simulink model "ROPOD_4Wheel_kinb_cntr"  (R2017b)
settings: Solver=FixedStepAuto  StartTime=0.0  StopTime=Inf  FixedStep=Ts  RelTol=1e-3
PreLoadFcn:
  | init_model
InitFcn:
  | init_model
values from neighbouring files (symbols this model uses):
  max_ropod_acc_theta = pi/16    (= 0.196349540849)    [init_model.m]
  max_ropod_acc_xy = 1.0    (= 1)    [init_model.m]
  max_ropod_vel_theta = pi/4    (= 0.785398163397)    [init_model.m]
  max_ropod_vel_xy = 1.5    [init_model.m]
  max_sw_current = 10    [init_model.m]
  Nwheels = 4    [init_model.m]
  pivot_offs_sws = [1.0998 0.2956 3.507 0.3641]    [init_model.m]
  SW_COM1_ENABLE1 = hex2dec('0001')    [init_model.m]
  SW_COM1_ENABLE2 = hex2dec('0002')    [init_model.m]
  SW_COM1_MODE_VELOCITY = bitshift(hex2dec('0002'),2)    [init_model.m]
  SW_COM1_USE_TS = hex2dec('8000')    [init_model.m]
  Ts = 0.001    [init_model.m]
  Tsp = 1    [init_model.m]
undefined symbols (not defined in the file or in its folder): Angular, CW1_1, CW1_2, CW1_3, CW1_4, CW2_1, CW2_2, CW2_3, CW2_4, d_w, DiscIntNeverNeededParam, Linear, Pose, ropod_kinmodel_param, rW1_1, rW1_2, rW1_3, rW1_4, rW2_1, rW2_2, rW2_3, rW2_4, s_w, Twist
libraries: robotlib x65, simulink x10, SOEM_EtherCAT_Lib x5, robotcorelib x1
(part 1 of 2)
PreSaveFcn:
  | init_model
settings Model: Creator=cesar  LastModifiedBy=cesar
settings OptimizationCC: PassReuseOutputArgsAs=Individual arguments  MaxStackSize=64
settings DebuggingCC: ParameterTunabilityLossMsg=error
settings HardwareCC: ProdBitPerLong=64  ProdHWDeviceType=Intel->x86-64 (Linux 64)  TargetBitPerLong=64  TargetBitPerPointer=64  TargetBitPerSizeT=64  TargetBitPerPtrDiffT=64  TargetLargestAtomicFloat=Float  TargetIntDivRoundTo=Zero  TargetEndianess=LittleEndian  TargetWordSize=64  TargetHWDeviceType=Intel->x86-64 (Linux 64)
settings SFSimCC: MATLABDynamicMemAlloc=off
settings RTWCC: SystemTargetFile=ert.tlc  HardwareBoard=Robot Operating System (ROS)  TemplateMakefile=ert_default_tmf  GenerateReport=on  RTWVerbose=off  CustomInclude=/usr/local/include/soem  CustomLibrary=/usr/local/lib/libsoem.so  Toolchain=Catkin  BuildConfiguration=Faster Runs  IncludeHyperlinkInReport=on  LaunchReport=on  TargetLang=C++  GenerateTraceInfo=on  GenerateTraceReport=on  GenerateTraceReportSl=on  GenerateTraceReportSf=on  GenerateTraceReportEml=on
settings CodeAppCC: ForceParamTrailComments=on  IgnoreCustomStorageClasses=off  OperatorAnnotations=on  SimulinkDataObjDesc=on  SFDataObjDesc=on  InsertBlockDesc=on
settings ERTTargetCC: SupportNonInlinedSFcns=on

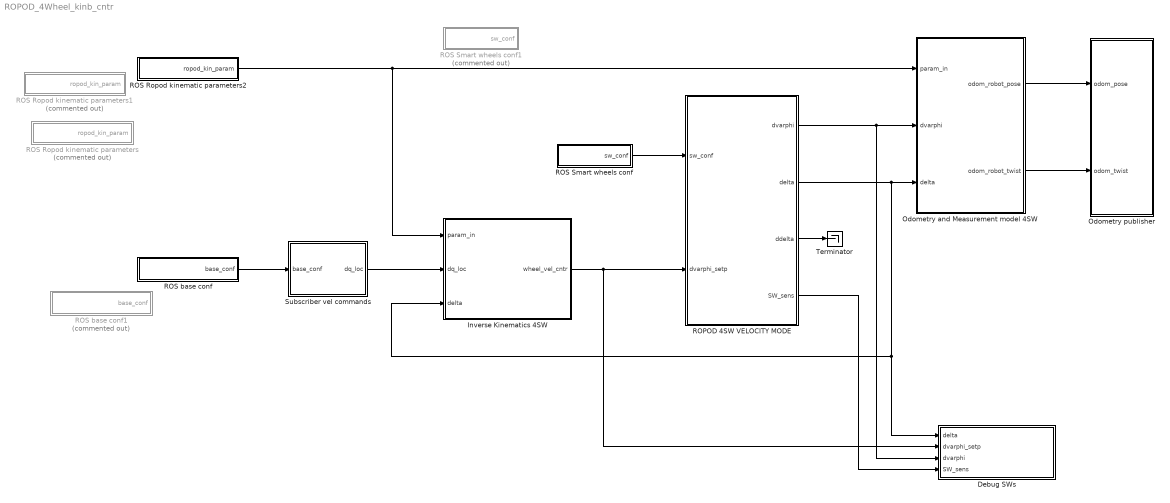
== system ROPOD_4Wheel_kinb_cntr ==
  Debug SWs : Subsystem
  Inverse Kinematics 4SW : Subsystem
  Odometry and Measurement model 4SW : Subsystem
  Odometry publisher : Subsystem
  ROPOD 4SW VELOCITY MODE : Subsystem
  ROS Ropod kinematic parameters : Subsystem  Commented=on
  ROS Ropod kinematic parameters1 : Subsystem  Commented=on
  ROS Ropod kinematic parameters2 : Subsystem
  ROS Smart wheels conf : Subsystem
  ROS Smart wheels conf1 : Subsystem  Commented=on
  ROS base conf : Subsystem
  ROS base conf1 : Subsystem  Commented=on
  Subscriber vel commands : Subsystem
  Terminator : Terminator
  wires:
  ROS Smart wheels conf/1(sw_conf) -> ROPOD 4SW VELOCITY MODE/1(sw_conf)
  ROS Ropod kinematic parameters2/1(ropod_kin_param) -> Inverse Kinematics 4SW/1(param_in), Odometry and Measurement model 4SW/1(param_in)
  Inverse Kinematics 4SW/1(wheel_vel_cntr) -> ROPOD 4SW VELOCITY MODE/2(dvarphi_setp), Debug SWs/2(dvarphi_setp)
  Odometry and Measurement model 4SW/1(odom_robot_pose) -> Odometry publisher/1(odom_pose)
  Odometry and Measurement model 4SW/2(odom_robot_twist) -> Odometry publisher/2(odom_twist)
  Subscriber vel commands/1(dq_loc) -> Inverse Kinematics 4SW/2(dq_loc)
  ROS base conf/1(base_conf) -> Subscriber vel commands/1(base_conf)
  ROPOD 4SW VELOCITY MODE/3(ddelta) -> Terminator/1
  ROPOD 4SW VELOCITY MODE/1(dvarphi) -> Odometry and Measurement model 4SW/2(dvarphi), Debug SWs/3(dvarphi)
  ROPOD 4SW VELOCITY MODE/2(delta) -> Inverse Kinematics 4SW/3(delta), Debug SWs/1(delta), Odometry and Measurement model 4SW/3(delta)
  ROPOD 4SW VELOCITY MODE/4(SW_sens) -> Debug SWs/4(SW_sens)

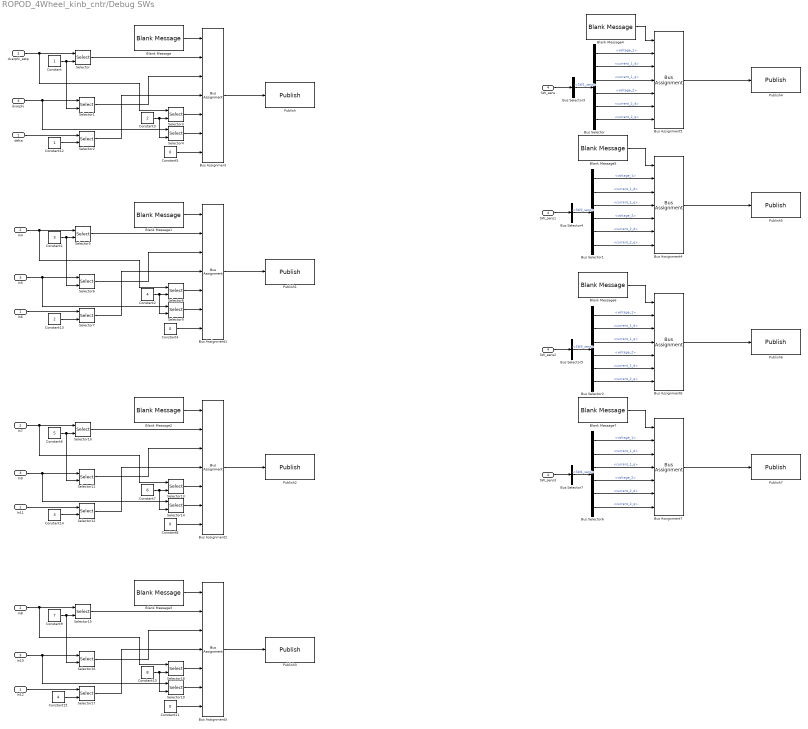
== system ROPOD_4Wheel_kinb_cntr/Debug SWs ==
  delta : Inport
  dvarphi_setp : Inport  Port=2
  dvarphi : Inport  Port=3
  SW_sens : Inport  Port=4
  Blank Message{,1..7} (8 alike) : robotlib/Blank Message  SourceLibraryInfo=This block requires Robotics System Toolbox  messageType=geometry_msgs/Twist  SampleTime=-1
      settings: SourceProductBaseCode=RO
  Bus Assignment{,1..7} (8 alike) : BusAssignment  AssignedSignals=Linear.X,Linear.Y,Linear.Z,Angular.X,Angular.Y,Angular.Z
  Bus Selector{,1..2,6} (4 alike) : BusSelector  OutputSignals=voltage_1,current_1_d,current_1_q,voltage_2,current_2_d,current_2_q
  Bus Selector3 : BusSelector  OutputSignals=SW1_sens
  Bus Selector4 : BusSelector  OutputSignals=SW2_sens
  Bus Selector5 : BusSelector  OutputSignals=SW3_sens
  Bus Selector7 : BusSelector  OutputSignals=SW4_sens
  Constant : Constant
  Constant1 : Constant  Value=3
  Constant10 : Constant  Value=8
  Constant{4..5,8,11} (4 alike) : Constant  Value=0
  Constant12 : Constant
  Constant13 : Constant  Value=2
  Constant14 : Constant  Value=3
  Constant15 : Constant  Value=4
  Constant2 : Constant  Value=4
  Constant3 : Constant  Value=2
  Constant6 : Constant  Value=5
  Constant7 : Constant  Value=6
  Constant9 : Constant  Value=7
  In10 : InportShadow  Port=3
  In11 : InportShadow
  In12 : InportShadow
  In4 : InportShadow  Port=2
  In5 : InportShadow  Port=3
  In6 : InportShadow
  In7 : InportShadow  Port=2
  In8 : InportShadow  Port=2
  In9 : InportShadow  Port=3
  Publish : robotlib/Publish  SourceLibraryInfo=This block requires Robotics System Toolbox  topicSource=Specify your own  topic=/smartw1_debug  messageType=geometry_msgs/Twist  messageQueueLength=1
      settings: SourceProductBaseCode=RO
  Publish1 : robotlib/Publish  SourceLibraryInfo=This block requires Robotics System Toolbox  topicSource=Specify your own  topic=/smartw2_debug  messageType=geometry_msgs/Twist  messageQueueLength=1
      settings: SourceProductBaseCode=RO
  Publish2 : robotlib/Publish  SourceLibraryInfo=This block requires Robotics System Toolbox  topicSource=Specify your own  topic=/smartw3_debug  messageType=geometry_msgs/Twist  messageQueueLength=1
      settings: SourceProductBaseCode=RO
  Publish3 : robotlib/Publish  SourceLibraryInfo=This block requires Robotics System Toolbox  topicSource=Specify your own  topic=/smartw4_debug  messageType=geometry_msgs/Twist  messageQueueLength=1
      settings: SourceProductBaseCode=RO
  Publish4 : robotlib/Publish  SourceLibraryInfo=This block requires Robotics System Toolbox  topicSource=Specify your own  topic=/smartw1_volcurr_debug  messageType=geometry_msgs/Twist  messageQueueLength=1
      settings: SourceProductBaseCode=RO
  Publish5 : robotlib/Publish  SourceLibraryInfo=This block requires Robotics System Toolbox  topicSource=Specify your own  topic=/smartw2_volcurr_debug  messageType=geometry_msgs/Twist  messageQueueLength=1
      settings: SourceProductBaseCode=RO
  Publish6 : robotlib/Publish  SourceLibraryInfo=This block requires Robotics System Toolbox  topicSource=Specify your own  topic=/smartw3_volcurr_debug  messageType=geometry_msgs/Twist  messageQueueLength=1
      settings: SourceProductBaseCode=RO
  Publish7 : robotlib/Publish  SourceLibraryInfo=This block requires Robotics System Toolbox  topicSource=Specify your own  topic=/smartw4_volcurr_debug  messageType=geometry_msgs/Twist  messageQueueLength=1
      settings: SourceProductBaseCode=RO
  SW_sens1 : InportShadow  Port=4
  SW_sens2 : InportShadow  Port=4
  SW_sens3 : InportShadow  Port=4
  Selector{,1,3..6,8..11,13..16,18..19} (16 alike) : Selector  InputPortWidth=8  IndexOptions=Index vector (port)  Indices=[1 3]  OutputSizes=1
  Selector{2,7,12,17} (4 alike) : Selector  InputPortWidth=4  IndexOptions=Index vector (port)  Indices=[1 3]  OutputSizes=1
  wires:
  delta/1 -> Selector2/1
  Constant5/1 -> Bus Assignment/7
  Selector2/1 -> Bus Assignment/4
  Selector3/1 -> Bus Assignment/5
  Constant/1 -> Selector1/2, Selector/2
  Blank Message/1 -> Bus Assignment/1
  Constant3/1 -> Selector4/2, Selector3/2
  Selector/1 -> Bus Assignment/2
  Selector1/1 -> Bus Assignment/3
  dvarphi/1 -> Selector4/1, Selector1/1
  Selector4/1 -> Bus Assignment/6
  dvarphi_setp/1 -> Selector3/1, Selector/1
  Bus Assignment/1 -> Publish/1
  Selector5/1 -> Bus Assignment1/2
  Blank Message1/1 -> Bus Assignment1/1
  Bus Assignment1/1 -> Publish1/1
  Selector7/1 -> Bus Assignment1/4
  In6/1 -> Selector7/1
  Constant2/1 -> Selector9/2, Selector8/2
  Constant1/1 -> Selector6/2, Selector5/2
  Selector8/1 -> Bus Assignment1/5
  Constant4/1 -> Bus Assignment1/7
  Selector6/1 -> Bus Assignment1/3
  Selector9/1 -> Bus Assignment1/6
  In4/1 -> Selector8/1, Selector5/1
  In5/1 -> Selector9/1, Selector6/1
  In11/1 -> Selector12/1
  Selector14/1 -> Bus Assignment2/6
  In9/1 -> Selector14/1, Selector11/1
  Blank Message2/1 -> Bus Assignment2/1
  Selector13/1 -> Bus Assignment2/5
  Constant7/1 -> Selector14/2, Selector13/2
  Selector12/1 -> Bus Assignment2/4
  Selector11/1 -> Bus Assignment2/3
  Constant6/1 -> Selector11/2, Selector10/2
  Bus Assignment2/1 -> Publish2/1
  Selector10/1 -> Bus Assignment2/2
  In7/1 -> Selector13/1, Selector10/1
  Constant8/1 -> Bus Assignment2/7
  In8/1 -> Selector18/1, Selector15/1
  Selector15/1 -> Bus Assignment3/2
  Selector19/1 -> Bus Assignment3/6
  Selector17/1 -> Bus Assignment3/4
  Selector16/1 -> Bus Assignment3/3
  Selector18/1 -> Bus Assignment3/5
  In10/1 -> Selector19/1, Selector16/1
  Constant9/1 -> Selector16/2, Selector15/2
  In12/1 -> Selector17/1
  Constant10/1 -> Selector19/2, Selector18/2
  Blank Message3/1 -> Bus Assignment3/1
  Constant11/1 -> Bus Assignment3/7
  Bus Assignment3/1 -> Publish3/1
  Constant12/1 -> Selector2/2
  Constant13/1 -> Selector7/2
  Constant14/1 -> Selector12/2
  Constant15/1 -> Selector17/2
  Bus Assignment5/1 -> Publish4/1
  Blank Message4/1 -> Bus Assignment5/1
  Bus Selector/2 -> Bus Assignment5/3  "<current_1_d>"
  Bus Selector/1 -> Bus Assignment5/2  "<voltage_1>"
  Bus Selector/3 -> Bus Assignment5/4  "<current_1_q>"
  Bus Selector/4 -> Bus Assignment5/5  "<voltage_2>"
  Bus Selector/5 -> Bus Assignment5/6  "<current_2_d>"
  Bus Selector/6 -> Bus Assignment5/7  "<current_2_q>"
  Bus Assignment4/1 -> Publish5/1
  Bus Selector1/3 -> Bus Assignment4/4  "<current_1_q>"
  Blank Message5/1 -> Bus Assignment4/1
  Bus Selector1/5 -> Bus Assignment4/6  "<current_2_d>"
  Bus Selector1/6 -> Bus Assignment4/7  "<current_2_q>"
  Bus Selector1/4 -> Bus Assignment4/5  "<voltage_2>"
  Bus Selector1/1 -> Bus Assignment4/2  "<voltage_1>"
  Bus Selector1/2 -> Bus Assignment4/3  "<current_1_d>"
  Bus Selector2/5 -> Bus Assignment6/6  "<current_2_d>"
  Bus Selector2/1 -> Bus Assignment6/2  "<voltage_1>"
  Bus Selector2/2 -> Bus Assignment6/3  "<current_1_d>"
  Bus Selector2/4 -> Bus Assignment6/5  "<voltage_2>"
  Bus Selector2/3 -> Bus Assignment6/4  "<current_1_q>"
  Bus Selector2/6 -> Bus Assignment6/7  "<current_2_q>"
  Bus Assignment6/1 -> Publish6/1
  Blank Message6/1 -> Bus Assignment6/1
  SW_sens/1 -> Bus Selector3/1
  Bus Selector3/1 -> Bus Selector/1  "<SW1_sens>"
  Bus Selector4/1 -> Bus Selector1/1  "<SW2_sens>"
  SW_sens1/1 -> Bus Selector4/1
  Bus Selector5/1 -> Bus Selector2/1  "<SW3_sens>"
  SW_sens2/1 -> Bus Selector5/1
  SW_sens3/1 -> Bus Selector7/1
  Bus Selector7/1 -> Bus Selector6/1  "<SW4_sens>"
  Blank Message7/1 -> Bus Assignment7/1
  Bus Assignment7/1 -> Publish7/1
  Bus Selector6/6 -> Bus Assignment7/7  "<current_2_q>"
  Bus Selector6/3 -> Bus Assignment7/4  "<current_1_q>"
  Bus Selector6/4 -> Bus Assignment7/5  "<voltage_2>"
  Bus Selector6/2 -> Bus Assignment7/3  "<current_1_d>"
  Bus Selector6/1 -> Bus Assignment7/2  "<voltage_1>"
  Bus Selector6/5 -> Bus Assignment7/6  "<current_2_d>"

== system ROPOD_4Wheel_kinb_cntr/Inverse Kinematics 4SW ==
  param_in : Inport
  dq_loc : Inport  Port=2
  delta : Inport  Port=3
  Gl_matrix : MATLAB Function  TreatAsAtomicUnit=on
  Product3 : Product  Multiplication=Matrix(*)
  Selector2 : Selector  InputPortWidth=3+3*Nwheels  IndexOptions=Index vector (dialog)  Indices=[3+Nwheels+1:3+3*Nwheels]  OutputSizes=1
  wheel_vel_cntr : Outport
  wires:
  param_in/1 -> Gl_matrix/1(ropod_kinmodel_param_vec)
  Gl_matrix/1(Gl) -> Product3/1
  Product3/1 -> Selector2/1
  delta/1 -> Gl_matrix/2(delta)
  dq_loc/1 -> Product3/2
  Selector2/1 -> wheel_vel_cntr/1

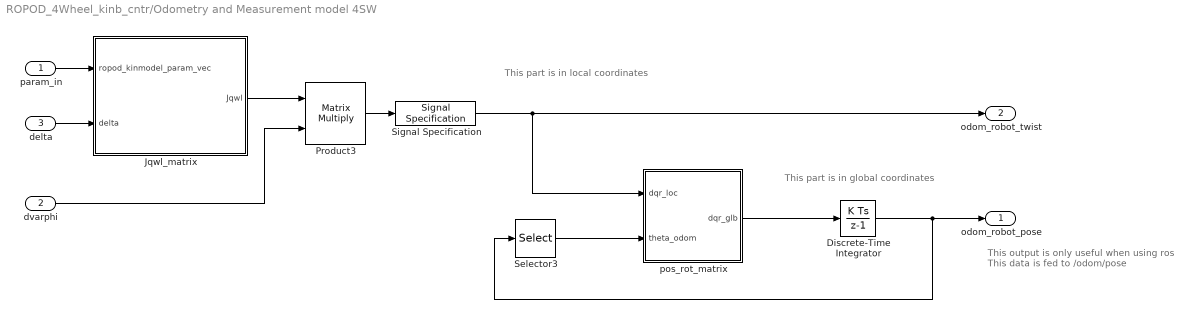
== system ROPOD_4Wheel_kinb_cntr/Odometry and Measurement model 4SW ==
  note: This output is only useful when using ros
      | This data is fed to /odom/pose
  note: This part is in global coordinates
  note: This part is in local coordinates
  param_in : Inport
  dvarphi : Inport  Port=2
  delta : Inport  Port=3
  Discrete-Time Integrator : DiscreteIntegrator  InitialConditionSetting=State (most efficient)  SampleTime=Ts  ICPrevOutput=DiscIntNeverNeededParam  ICPrevScaledInput=DiscIntNeverNeededParam
  Jqwl_matrix : MATLAB Function  TreatAsAtomicUnit=on
  Product3 : Product  Multiplication=Matrix(*)
  Selector3 : Selector  InputPortWidth=3  IndexOptions=Index vector (dialog)  Indices=3  OutputSizes=1
  Signal Specification : SignalSpecification  Dimensions=[3 1]
  pos_rot_matrix : MATLAB Function  TreatAsAtomicUnit=on
  odom_robot_pose : Outport
  odom_robot_twist : Outport  Port=2
  wires:
  Product3/1 -> Signal Specification/1
  param_in/1 -> Jqwl_matrix/1(ropod_kinmodel_param_vec)
  delta/1 -> Jqwl_matrix/2(delta)
  Jqwl_matrix/1(Jqwl) -> Product3/1
  dvarphi/1 -> Product3/2
  Signal Specification/1 -> pos_rot_matrix/1(dqr_loc), odom_robot_twist/1
  Selector3/1 -> pos_rot_matrix/2(theta_odom)
  pos_rot_matrix/1(dqr_glb) -> Discrete-Time Integrator/1
  Discrete-Time Integrator/1 -> odom_robot_pose/1, Selector3/1

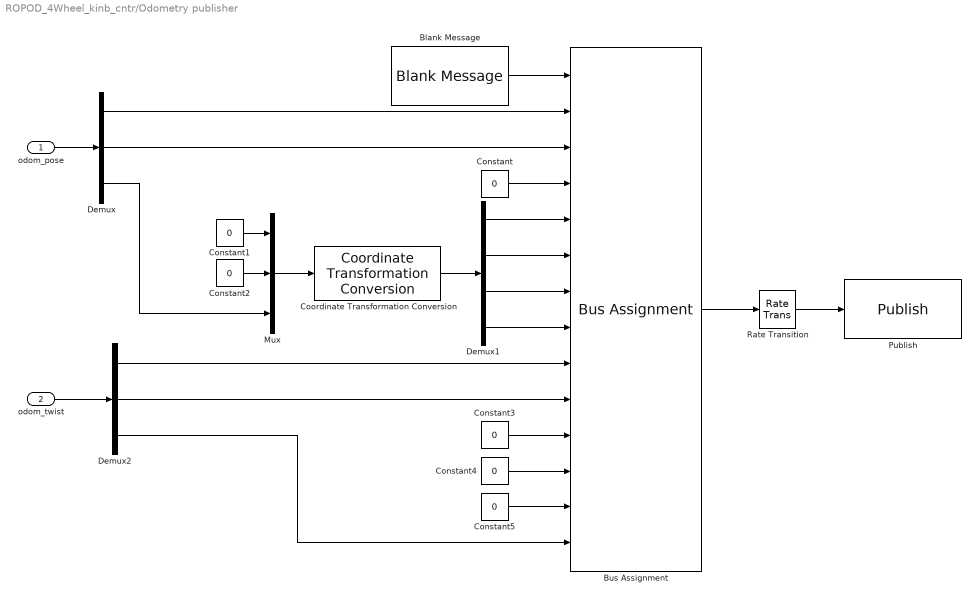
== system ROPOD_4Wheel_kinb_cntr/Odometry publisher ==
  odom_pose : Inport
  odom_twist : Inport  Port=2
  Blank Message : robotlib/Blank Message  SourceLibraryInfo=This block requires Robotics System Toolbox  messageType=nav_msgs/Odometry  SampleTime=-1
      settings: SourceProductBaseCode=RO
  Bus Assignment : BusAssignment  AssignedSignals=Pose.Pose.Position.X,Pose.Pose.Position.Y,Pose.Pose.Position.Z,Pose.Pose.Orientation.X,Pose.Pose.Orientation.Y,Pose.Pose.Orientation.Z,Pose.Pose.Orientation.W,Twist.Twist.Linear.X,Twist.Twist.Linear.Y,Twist.Twist.Linear.Z,Twist.Twist.Angular.X,Twist.Twist.Angular.Y,Twist.Twist.Angular.Z
  Constant{,1..5} (6 alike) : Constant  Value=0
  Coordinate Transformation Conversion : robotcorelib/Coordinate Transformation Conversion  InputRepresentation=Euler Angles  InputEulerSequence=XYZ  ShowTrVecInputPort=on  OutputRepresentation=Quaternion  OutputEulerSequence=ZYX  ShowTrVecOutputPort=on  SimulateUsing=Code generation
      settings: SourceProductBaseCode=RO
  Demux : Demux  Outputs=3
  Demux1 : Demux
  Demux2 : Demux  Outputs=3
  Mux : Mux  Inputs=3
  Publish : robotlib/Publish  SourceLibraryInfo=This block requires Robotics System Toolbox  topicSource=Specify your own  topic=/pico/odom  messageType=nav_msgs/Odometry  messageQueueLength=1
      settings: SourceProductBaseCode=RO
  Rate Transition : RateTransition  OutPortSampleTime=Ts_rost
  wires:
  Demux2/2 -> Bus Assignment/10
  Bus Assignment/1 -> Rate Transition/1
  Constant2/1 -> Mux/2
  Demux1/2 -> Bus Assignment/6
  Constant3/1 -> Bus Assignment/11
  Constant/1 -> Bus Assignment/4
  Constant4/1 -> Bus Assignment/12
  Demux2/1 -> Bus Assignment/9
  Coordinate Transformation Conversion/1 -> Demux1/1
  Constant5/1 -> Bus Assignment/13
  Demux/3 -> Mux/3
  Mux/1 -> Coordinate Transformation Conversion/1
  Demux1/3 -> Bus Assignment/7
  odom_pose/1 -> Demux/1
  Demux1/1 -> Bus Assignment/5
  Demux/1 -> Bus Assignment/2
  Demux1/4 -> Bus Assignment/8
  Constant1/1 -> Mux/1
  odom_twist/1 -> Demux2/1
  Demux/2 -> Bus Assignment/3
  Blank Message/1 -> Bus Assignment/1
  Demux2/3 -> Bus Assignment/14
  Rate Transition/1 -> Publish/1

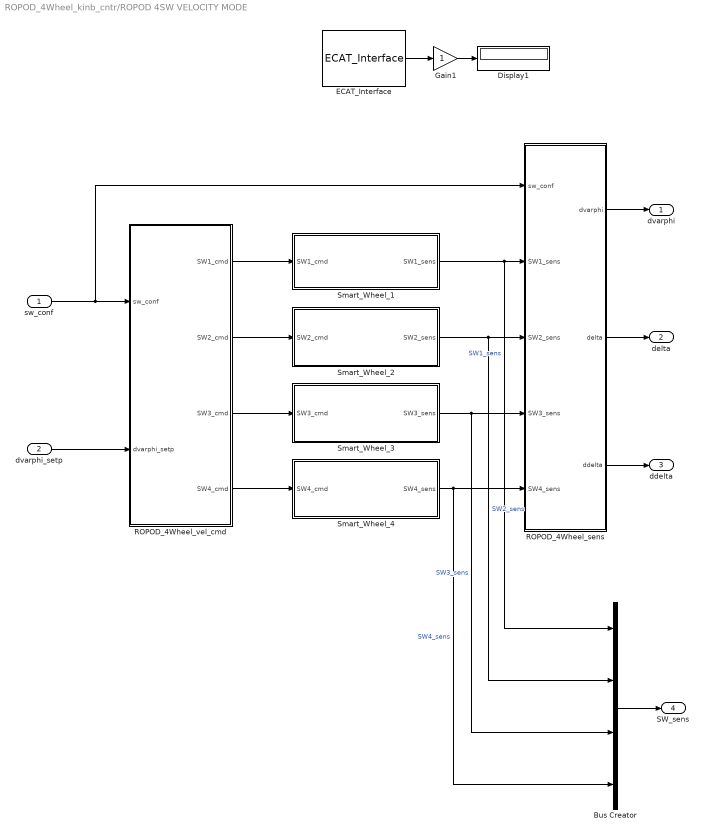
== system ROPOD_4Wheel_kinb_cntr/ROPOD 4SW VELOCITY MODE ==
  sw_conf : Inport
  dvarphi_setp : Inport  Port=2
  Bus Creator : BusCreator  Inputs=4
  Display1 : Display
  ECAT_Interface : SOEM_EtherCAT_Lib/ECAT_Interface  Priority=0  IFINTERFACE=eth0  TS=Ts
      settings: SourceProductName=SOEM_EtherCAT_Lib
  Gain1 : Gain  OutDataTypeStr=double
  ROPOD_4Wheel_sens : Subsystem
  ROPOD_4Wheel_vel_cmd : Subsystem
  Smart_Wheel_1 : Subsystem
  Smart_Wheel_2 : Subsystem
  Smart_Wheel_3 : Subsystem
  Smart_Wheel_4 : Subsystem
  dvarphi : Outport
  delta : Outport  Port=2
  ddelta : Outport  Port=3
  SW_sens : Outport  Port=4
  wires:
  dvarphi_setp/1 -> ROPOD_4Wheel_vel_cmd/2(dvarphi_setp)
  ROPOD_4Wheel_vel_cmd/2(SW2_cmd) -> Smart_Wheel_2/1(SW2_cmd)
  sw_conf/1 -> ROPOD_4Wheel_sens/1(sw_conf), ROPOD_4Wheel_vel_cmd/1(sw_conf)
  ROPOD_4Wheel_vel_cmd/1(SW1_cmd) -> Smart_Wheel_1/1(SW1_cmd)
  Smart_Wheel_1/1(SW1_sens) -> Bus Creator/1, ROPOD_4Wheel_sens/2(SW1_sens)  "SW1_sens"
  ROPOD_4Wheel_sens/2(delta) -> delta/1
  ROPOD_4Wheel_sens/1(dvarphi) -> dvarphi/1
  ECAT_Interface/1 -> Gain1/1
  Gain1/1 -> Display1/1
  ROPOD_4Wheel_vel_cmd/3(SW3_cmd) -> Smart_Wheel_3/1(SW3_cmd)
  ROPOD_4Wheel_sens/3(ddelta) -> ddelta/1
  ROPOD_4Wheel_vel_cmd/4(SW4_cmd) -> Smart_Wheel_4/1(SW4_cmd)
  Smart_Wheel_2/1(SW2_sens) -> Bus Creator/2, ROPOD_4Wheel_sens/3(SW2_sens)  "SW2_sens"
  Smart_Wheel_3/1(SW3_sens) -> Bus Creator/3, ROPOD_4Wheel_sens/4(SW3_sens)  "SW3_sens"
  Smart_Wheel_4/1(SW4_sens) -> Bus Creator/4, ROPOD_4Wheel_sens/5(SW4_sens)  "SW4_sens"
  Bus Creator/1 -> SW_sens/1

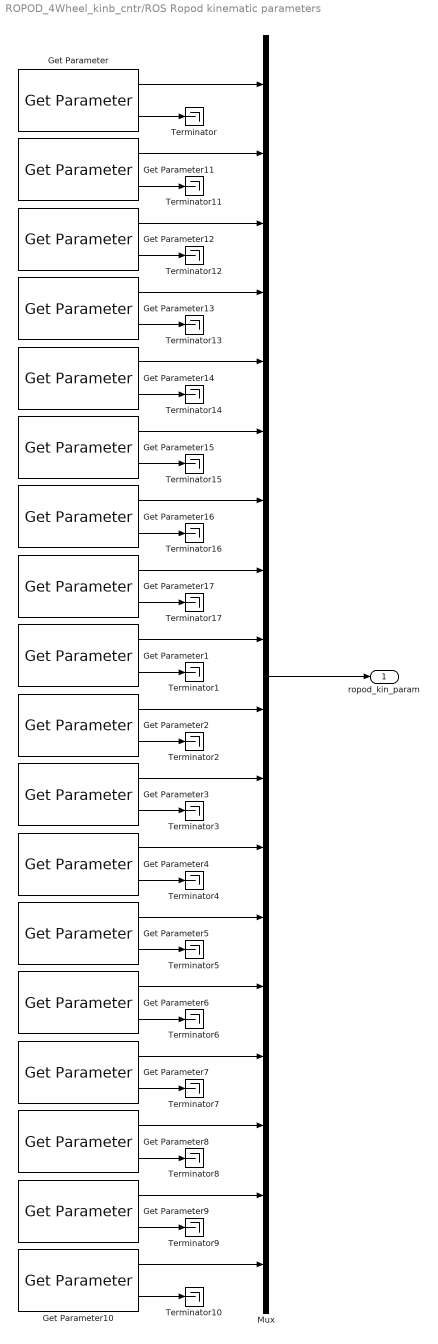
== system ROPOD_4Wheel_kinb_cntr/ROS Ropod kinematic parameters ==
  Get Parameter : robotlib/Get Parameter  SourceLibraryInfo=This block requires Robotics System Toolbox  ParameterSource=Specify your own  ParameterName=/base_kin_model/r_wL_SW1  ParameterType=double  ParameterMaxArrayLength=16  ParameterInitialValue=ropod_kinmodel_param.r_w(1)  SampleTime=-1  ShowErrorCodeOutput=on  ModelName=ROPOD_4Wheel_kinb_cntr  BlockId=ParamGet_ROPOD_4Wheel_kinb_cntr_466
      settings: SourceProductName=Robotics System Toolbox  SourceProductBaseCode=RO
  Get Parameter1 : robotlib/Get Parameter  SourceLibraryInfo=This block requires Robotics System Toolbox  ParameterSource=Specify your own  ParameterName=/base_kin_model/s_w  ParameterType=double  ParameterMaxArrayLength=16  ParameterInitialValue=ropod_kinmodel_param.s_w  SampleTime=-1  ShowErrorCodeOutput=on  ModelName=ROPOD_4Wheel_kinb_cntr  BlockId=ParamGet_ROPOD_4Wheel_kinb_cntr_470
      settings: SourceProductName=Robotics System Toolbox  SourceProductBaseCode=RO
  Get Parameter10 : robotlib/Get Parameter  SourceLibraryInfo=This block requires Robotics System Toolbox  ParameterSource=Specify your own  ParameterName=/base_kin_model/ypos_SW4  ParameterType=double  ParameterMaxArrayLength=16  ParameterInitialValue=ropod_kinmodel_param.C_SW(8)  SampleTime=-1  ShowErrorCodeOutput=on  ModelName=ROPOD_4Wheel_kinb_cntr  BlockId=ParamGet_ROPOD_4Wheel_kinb_cntr_617
      settings: SourceProductName=Robotics System Toolbox  SourceProductBaseCode=RO
  Get Parameter11 : robotlib/Get Parameter  SourceLibraryInfo=This block requires Robotics System Toolbox  ParameterSource=Specify your own  ParameterName=/base_kin_model/r_wR_SW1  ParameterType=double  ParameterMaxArrayLength=16  ParameterInitialValue=ropod_kinmodel_param.r_w(2)  SampleTime=-1  ShowErrorCodeOutput=on  ModelName=ROPOD_4Wheel_kinb_cntr  BlockId=ParamGet_ROPOD_4Wheel_kinb_cntr_648
      settings: SourceProductName=Robotics System Toolbox  SourceProductBaseCode=RO
  Get Parameter12 : robotlib/Get Parameter  SourceLibraryInfo=This block requires Robotics System Toolbox  ParameterSource=Specify your own  ParameterName=/base_kin_model/r_wL_SW2  ParameterType=double  ParameterMaxArrayLength=16  ParameterInitialValue=ropod_kinmodel_param.r_w(3)  SampleTime=-1  ShowErrorCodeOutput=on  ModelName=ROPOD_4Wheel_kinb_cntr  BlockId=ParamGet_ROPOD_4Wheel_kinb_cntr_650
      settings: SourceProductName=Robotics System Toolbox  SourceProductBaseCode=RO
  Get Parameter13 : robotlib/Get Parameter  SourceLibraryInfo=This block requires Robotics System Toolbox  ParameterSource=Specify your own  ParameterName=/base_kin_model/r_wR_SW2  ParameterType=double  ParameterMaxArrayLength=16  ParameterInitialValue=ropod_kinmodel_param.r_w(4)  SampleTime=-1  ShowErrorCodeOutput=on  ModelName=ROPOD_4Wheel_kinb_cntr  BlockId=ParamGet_ROPOD_4Wheel_kinb_cntr_651
      settings: SourceProductName=Robotics System Toolbox  SourceProductBaseCode=RO
  Get Parameter14 : robotlib/Get Parameter  SourceLibraryInfo=This block requires Robotics System Toolbox  ParameterSource=Specify your own  ParameterName=/base_kin_model/r_wL_SW3  ParameterType=double  ParameterMaxArrayLength=16  ParameterInitialValue=ropod_kinmodel_param.r_w(5)  SampleTime=-1  ShowErrorCodeOutput=on  ModelName=ROPOD_4Wheel_kinb_cntr  BlockId=ParamGet_ROPOD_4Wheel_kinb_cntr_654
      settings: SourceProductName=Robotics System Toolbox  SourceProductBaseCode=RO
  Get Parameter15 : robotlib/Get Parameter  SourceLibraryInfo=This block requires Robotics System Toolbox  ParameterSource=Specify your own  ParameterName=/base_kin_model/r_wR_SW3  ParameterType=double  ParameterMaxArrayLength=16  ParameterInitialValue=ropod_kinmodel_param.r_w(6)  SampleTime=-1  ShowErrorCodeOutput=on  ModelName=ROPOD_4Wheel_kinb_cntr  BlockId=ParamGet_ROPOD_4Wheel_kinb_cntr_655
      settings: SourceProductName=Robotics System Toolbox  SourceProductBaseCode=RO
  Get Parameter16 : robotlib/Get Parameter  SourceLibraryInfo=This block requires Robotics System Toolbox  ParameterSource=Specify your own  ParameterName=/base_kin_model/r_wL_SW4  ParameterType=double  ParameterMaxArrayLength=16  ParameterInitialValue=ropod_kinmodel_param.r_w(7)  SampleTime=-1  ShowErrorCodeOutput=on  ModelName=ROPOD_4Wheel_kinb_cntr  BlockId=ParamGet_ROPOD_4Wheel_kinb_cntr_656
      settings: SourceProductName=Robotics System Toolbox  SourceProductBaseCode=RO
  Get Parameter17 : robotlib/Get Parameter  SourceLibraryInfo=This block requires Robotics System Toolbox  ParameterSource=Specify your own  ParameterName=/base_kin_model/r_wR_SW4  ParameterType=double  ParameterMaxArrayLength=16  ParameterInitialValue=ropod_kinmodel_param.r_w(8)  SampleTime=-1  ShowErrorCodeOutput=on  ModelName=ROPOD_4Wheel_kinb_cntr  BlockId=ParamGet_ROPOD_4Wheel_kinb_cntr_657
      settings: SourceProductName=Robotics System Toolbox  SourceProductBaseCode=RO
  Get Parameter2 : robotlib/Get Parameter  SourceLibraryInfo=This block requires Robotics System Toolbox  ParameterSource=Specify your own  ParameterName=/base_kin_model/d_w  ParameterType=double  ParameterMaxArrayLength=16  ParameterInitialValue=ropod_kinmodel_param.d_w  SampleTime=-1  ShowErrorCodeOutput=on  ModelName=ROPOD_4Wheel_kinb_cntr  BlockId=ParamGet_ROPOD_4Wheel_kinb_cntr_472
      settings: SourceProductName=Robotics System Toolbox  SourceProductBaseCode=RO
  Get Parameter3 : robotlib/Get Parameter  SourceLibraryInfo=This block requires Robotics System Toolbox  ParameterSource=Specify your own  ParameterName=/base_kin_model/xpos_SW1  ParameterType=double  ParameterMaxArrayLength=16  ParameterInitialValue=ropod_kinmodel_param.C_SW(1)  SampleTime=-1  ShowErrorCodeOutput=on  ModelName=ROPOD_4Wheel_kinb_cntr  BlockId=ParamGet_ROPOD_4Wheel_kinb_cntr_473
      settings: SourceProductName=Robotics System Toolbox  SourceProductBaseCode=RO
  Get Parameter4 : robotlib/Get Parameter  SourceLibraryInfo=This block requires Robotics System Toolbox  ParameterSource=Specify your own  ParameterName=/base_kin_model/ypos_SW1  ParameterType=double  ParameterMaxArrayLength=16  ParameterInitialValue=ropod_kinmodel_param.C_SW(2)  SampleTime=-1  ShowErrorCodeOutput=on  ModelName=ROPOD_4Wheel_kinb_cntr  BlockId=ParamGet_ROPOD_4Wheel_kinb_cntr_474
      settings: SourceProductName=Robotics System Toolbox  SourceProductBaseCode=RO
  Get Parameter5 : robotlib/Get Parameter  SourceLibraryInfo=This block requires Robotics System Toolbox  ParameterSource=Specify your own  ParameterName=/base_kin_model/xpos_SW2  ParameterType=double  ParameterMaxArrayLength=16  ParameterInitialValue=ropod_kinmodel_param.C_SW(3)  SampleTime=-1  ShowErrorCodeOutput=on  ModelName=ROPOD_4Wheel_kinb_cntr  BlockId=ParamGet_ROPOD_4Wheel_kinb_cntr_475
      settings: SourceProductName=Robotics System Toolbox  SourceProductBaseCode=RO
  Get Parameter6 : robotlib/Get Parameter  SourceLibraryInfo=This block requires Robotics System Toolbox  ParameterSource=Specify your own  ParameterName=/base_kin_model/ypos_SW2  ParameterType=double  ParameterMaxArrayLength=16  ParameterInitialValue=ropod_kinmodel_param.C_SW(4)  SampleTime=-1  ShowErrorCodeOutput=on  ModelName=ROPOD_4Wheel_kinb_cntr  BlockId=ParamGet_ROPOD_4Wheel_kinb_cntr_476
      settings: SourceProductName=Robotics System Toolbox  SourceProductBaseCode=RO
  Get Parameter7 : robotlib/Get Parameter  SourceLibraryInfo=This block requires Robotics System Toolbox  ParameterSource=Specify your own  ParameterName=/base_kin_model/xpos_SW3  ParameterType=double  ParameterMaxArrayLength=16  ParameterInitialValue=ropod_kinmodel_param.C_SW(5)  SampleTime=-1  ShowErrorCodeOutput=on  ModelName=ROPOD_4Wheel_kinb_cntr  BlockId=ParamGet_ROPOD_4Wheel_kinb_cntr_559
      settings: SourceProductName=Robotics System Toolbox  SourceProductBaseCode=RO
  Get Parameter8 : robotlib/Get Parameter  SourceLibraryInfo=This block requires Robotics System Toolbox  ParameterSource=Specify your own  ParameterName=/base_kin_model/ypos_SW3  ParameterType=double  ParameterMaxArrayLength=16  ParameterInitialValue=ropod_kinmodel_param.C_SW(6)  SampleTime=-1  ShowErrorCodeOutput=on  ModelName=ROPOD_4Wheel_kinb_cntr  BlockId=ParamGet_ROPOD_4Wheel_kinb_cntr_560
      settings: SourceProductName=Robotics System Toolbox  SourceProductBaseCode=RO
  Get Parameter9 : robotlib/Get Parameter  SourceLibraryInfo=This block requires Robotics System Toolbox  ParameterSource=Specify your own  ParameterName=/base_kin_model/xpos_SW4  ParameterType=double  ParameterMaxArrayLength=16  ParameterInitialValue=ropod_kinmodel_param.C_SW(7)  SampleTime=-1  ShowErrorCodeOutput=on  ModelName=ROPOD_4Wheel_kinb_cntr  BlockId=ParamGet_ROPOD_4Wheel_kinb_cntr_616
      settings: SourceProductName=Robotics System Toolbox  SourceProductBaseCode=RO
  Mux : Mux  Inputs=18
  Terminator{,1..17} (18 alike) : Terminator
  ropod_kin_param : Outport
  wires:
  Get Parameter/2 -> Terminator/1
  Get Parameter1/2 -> Terminator1/1
  Get Parameter3/2 -> Terminator3/1
  Get Parameter2/2 -> Terminator2/1
  Get Parameter4/2 -> Terminator4/1
  Get Parameter5/2 -> Terminator5/1
  Get Parameter6/2 -> Terminator6/1
  Mux/1 -> ropod_kin_param/1
  Get Parameter7/2 -> Terminator7/1
  Get Parameter8/2 -> Terminator8/1
  Get Parameter10/2 -> Terminator10/1
  Get Parameter9/2 -> Terminator9/1
  Get Parameter11/2 -> Terminator11/1
  Get Parameter13/2 -> Terminator13/1
  Get Parameter12/2 -> Terminator12/1
  Get Parameter16/2 -> Terminator16/1
  Get Parameter17/2 -> Terminator17/1
  Get Parameter15/2 -> Terminator15/1
  Get Parameter14/2 -> Terminator14/1
  Get Parameter/1 -> Mux/1
  Get Parameter11/1 -> Mux/2
  Get Parameter12/1 -> Mux/3
  Get Parameter13/1 -> Mux/4
  Get Parameter14/1 -> Mux/5
  Get Parameter15/1 -> Mux/6
  Get Parameter16/1 -> Mux/7
  Get Parameter17/1 -> Mux/8
  Get Parameter1/1 -> Mux/9
  Get Parameter2/1 -> Mux/10
  Get Parameter3/1 -> Mux/11
  Get Parameter4/1 -> Mux/12
  Get Parameter5/1 -> Mux/13
  Get Parameter6/1 -> Mux/14
  Get Parameter7/1 -> Mux/15
  Get Parameter8/1 -> Mux/16
  Get Parameter9/1 -> Mux/17
  Get Parameter10/1 -> Mux/18

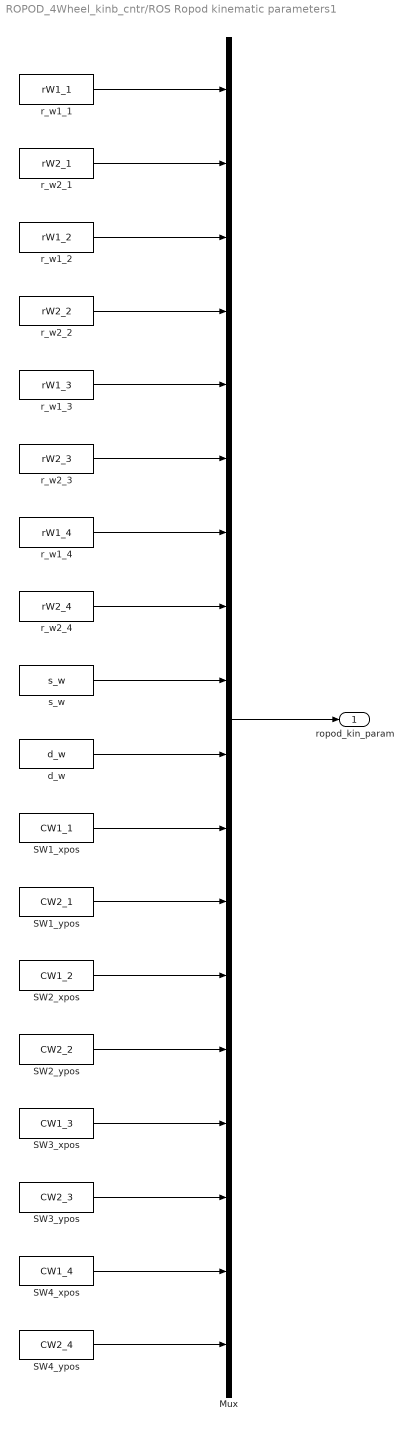
== system ROPOD_4Wheel_kinb_cntr/ROS Ropod kinematic parameters1 ==
  Mux : Mux  Inputs=18
  SW1_xpos : Constant  Value=CW1_1
  SW1_ypos : Constant  Value=CW2_1
  SW2_xpos : Constant  Value=CW1_2
  SW2_ypos : Constant  Value=CW2_2
  SW3_xpos : Constant  Value=CW1_3
  SW3_ypos : Constant  Value=CW2_3
  SW4_xpos : Constant  Value=CW1_4
  SW4_ypos : Constant  Value=CW2_4
  d_w : Constant  Value=d_w
  r_w1_1 : Constant  Value=rW1_1
  r_w1_2 : Constant  Value=rW1_2
  r_w1_3 : Constant  Value=rW1_3
  r_w1_4 : Constant  Value=rW1_4
  r_w2_1 : Constant  Value=rW2_1
  r_w2_2 : Constant  Value=rW2_2
  r_w2_3 : Constant  Value=rW2_3
  r_w2_4 : Constant  Value=rW2_4
  s_w : Constant  Value=s_w
  ropod_kin_param : Outport
  wires:
  Mux/1 -> ropod_kin_param/1
  r_w1_1/1 -> Mux/1
  r_w2_1/1 -> Mux/2
  r_w1_2/1 -> Mux/3
  r_w2_2/1 -> Mux/4
  r_w1_3/1 -> Mux/5
  r_w2_3/1 -> Mux/6
  r_w1_4/1 -> Mux/7
  r_w2_4/1 -> Mux/8
  s_w/1 -> Mux/9
  d_w/1 -> Mux/10
  SW1_xpos/1 -> Mux/11
  SW1_ypos/1 -> Mux/12
  SW2_xpos/1 -> Mux/13
  SW2_ypos/1 -> Mux/14
  SW3_xpos/1 -> Mux/15
  SW3_ypos/1 -> Mux/16
  SW4_xpos/1 -> Mux/17
  SW4_ypos/1 -> Mux/18

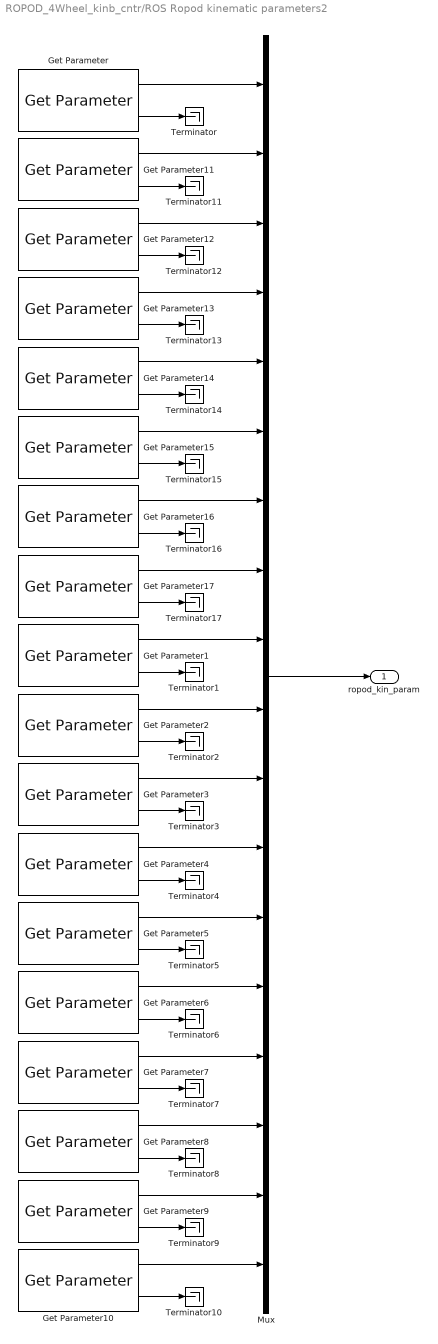
== system ROPOD_4Wheel_kinb_cntr/ROS Ropod kinematic parameters2 ==
  Get Parameter : robotlib/Get Parameter  SourceLibraryInfo=This block requires Robotics System Toolbox  ParameterSource=Specify your own  ParameterName=/base_kin_model/r_wL_SW1  ParameterType=double  ParameterMaxArrayLength=16  ParameterInitialValue=ropod_kinmodel_param.r_w(1)  SampleTime=Tsp  ShowErrorCodeOutput=on  ModelName=ROPOD_4Wheel_kinb_cntr  BlockId=ParamGet_ROPOD_4Wheel_kinb_cntr_1081
      settings: SourceProductName=Robotics System Toolbox  SourceProductBaseCode=RO
  Get Parameter1 : robotlib/Get Parameter  SourceLibraryInfo=This block requires Robotics System Toolbox  ParameterSource=Specify your own  ParameterName=/base_kin_model/s_w  ParameterType=double  ParameterMaxArrayLength=16  ParameterInitialValue=ropod_kinmodel_param.s_w  SampleTime=Tsp  ShowErrorCodeOutput=on  ModelName=ROPOD_4Wheel_kinb_cntr  BlockId=ParamGet_ROPOD_4Wheel_kinb_cntr_1097
      settings: SourceProductName=Robotics System Toolbox  SourceProductBaseCode=RO
  Get Parameter10 : robotlib/Get Parameter  SourceLibraryInfo=This block requires Robotics System Toolbox  ParameterSource=Specify your own  ParameterName=/base_kin_model/ypos_SW4  ParameterType=double  ParameterMaxArrayLength=16  ParameterInitialValue=ropod_kinmodel_param.C_SW(8)  SampleTime=Tsp  ShowErrorCodeOutput=on  ModelName=ROPOD_4Wheel_kinb_cntr  BlockId=ParamGet_ROPOD_4Wheel_kinb_cntr_1109
      settings: SourceProductName=Robotics System Toolbox  SourceProductBaseCode=RO
  Get Parameter11 : robotlib/Get Parameter  SourceLibraryInfo=This block requires Robotics System Toolbox  ParameterSource=Specify your own  ParameterName=/base_kin_model/r_wR_SW1  ParameterType=double  ParameterMaxArrayLength=16  ParameterInitialValue=ropod_kinmodel_param.r_w(2)  SampleTime=Tsp  ShowErrorCodeOutput=on  ModelName=ROPOD_4Wheel_kinb_cntr  BlockId=ParamGet_ROPOD_4Wheel_kinb_cntr_1082
      settings: SourceProductName=Robotics System Toolbox  SourceProductBaseCode=RO
  Get Parameter12 : robotlib/Get Parameter  SourceLibraryInfo=This block requires Robotics System Toolbox  ParameterSource=Specify your own  ParameterName=/base_kin_model/r_wL_SW2  ParameterType=double  ParameterMaxArrayLength=16  ParameterInitialValue=ropod_kinmodel_param.r_w(3)  SampleTime=Tsp  ShowErrorCodeOutput=on  ModelName=ROPOD_4Wheel_kinb_cntr  BlockId=ParamGet_ROPOD_4Wheel_kinb_cntr_1083
      settings: SourceProductName=Robotics System Toolbox  SourceProductBaseCode=RO
  Get Parameter13 : robotlib/Get Parameter  SourceLibraryInfo=This block requires Robotics System Toolbox  ParameterSource=Specify your own  ParameterName=/base_kin_model/r_wR_SW2  ParameterType=double  ParameterMaxArrayLength=16  ParameterInitialValue=ropod_kinmodel_param.r_w(4)  SampleTime=Tsp  ShowErrorCodeOutput=on  ModelName=ROPOD_4Wheel_kinb_cntr  BlockId=ParamGet_ROPOD_4Wheel_kinb_cntr_1084
      settings: SourceProductName=Robotics System Toolbox  SourceProductBaseCode=RO
  Get Parameter14 : robotlib/Get Parameter  SourceLibraryInfo=This block requires Robotics System Toolbox  ParameterSource=Specify your own  ParameterName=/base_kin_model/r_wL_SW3  ParameterType=double  ParameterMaxArrayLength=16  ParameterInitialValue=ropod_kinmodel_param.r_w(5)  SampleTime=Tsp  ShowErrorCodeOutput=on  ModelName=ROPOD_4Wheel_kinb_cntr  BlockId=ParamGet_ROPOD_4Wheel_kinb_cntr_1085
      settings: SourceProductName=Robotics System Toolbox  SourceProductBaseCode=RO
  Get Parameter15 : robotlib/Get Parameter  SourceLibraryInfo=This block requires Robotics System Toolbox  ParameterSource=Specify your own  ParameterName=/base_kin_model/r_wR_SW3  ParameterType=double  ParameterMaxArrayLength=16  ParameterInitialValue=ropod_kinmodel_param.r_w(6)  SampleTime=Tsp  ShowErrorCodeOutput=on  ModelName=ROPOD_4Wheel_kinb_cntr  BlockId=ParamGet_ROPOD_4Wheel_kinb_cntr_1086
      settings: SourceProductName=Robotics System Toolbox  SourceProductBaseCode=RO
  Get Parameter16 : robotlib/Get Parameter  SourceLibraryInfo=This block requires Robotics System Toolbox  ParameterSource=Specify your own  ParameterName=/base_kin_model/r_wL_SW4  ParameterType=double  ParameterMaxArrayLength=16  ParameterInitialValue=ropod_kinmodel_param.r_w(7)  SampleTime=Tsp  ShowErrorCodeOutput=on  ModelName=ROPOD_4Wheel_kinb_cntr  BlockId=ParamGet_ROPOD_4Wheel_kinb_cntr_1087
      settings: SourceProductName=Robotics System Toolbox  SourceProductBaseCode=RO
  Get Parameter17 : robotlib/Get Parameter  SourceLibraryInfo=This block requires Robotics System Toolbox  ParameterSource=Specify your own  ParameterName=/base_kin_model/r_wR_SW4  ParameterType=double  ParameterMaxArrayLength=16  ParameterInitialValue=ropod_kinmodel_param.r_w(8)  SampleTime=Tsp  ShowErrorCodeOutput=on  ModelName=ROPOD_4Wheel_kinb_cntr  BlockId=ParamGet_ROPOD_4Wheel_kinb_cntr_1088
      settings: SourceProductName=Robotics System Toolbox  SourceProductBaseCode=RO
  Get Parameter2 : robotlib/Get Parameter  SourceLibraryInfo=This block requires Robotics System Toolbox  ParameterSource=Specify your own  ParameterName=/base_kin_model/d_w  ParameterType=double  ParameterMaxArrayLength=16  ParameterInitialValue=ropod_kinmodel_param.d_w  SampleTime=Tsp  ShowErrorCodeOutput=on  ModelName=ROPOD_4Wheel_kinb_cntr  BlockId=ParamGet_ROPOD_4Wheel_kinb_cntr_1098
      settings: SourceProductName=Robotics System Toolbox  SourceProductBaseCode=RO
  Get Parameter3 : robotlib/Get Parameter  SourceLibraryInfo=This block requires Robotics System Toolbox  ParameterSource=Specify your own  ParameterName=/base_kin_model/xpos_SW1  ParameterType=double  ParameterMaxArrayLength=16  ParameterInitialValue=ropod_kinmodel_param.C_SW(1)  SampleTime=Tsp  ShowErrorCodeOutput=on  ModelName=ROPOD_4Wheel_kinb_cntr  BlockId=ParamGet_ROPOD_4Wheel_kinb_cntr_1101
      settings: SourceProductName=Robotics System Toolbox  SourceProductBaseCode=RO
  Get Parameter4 : robotlib/Get Parameter  SourceLibraryInfo=This block requires Robotics System Toolbox  ParameterSource=Specify your own  ParameterName=/base_kin_model/ypos_SW1  ParameterType=double  ParameterMaxArrayLength=16  ParameterInitialValue=ropod_kinmodel_param.C_SW(2)  SampleTime=Tsp  ShowErrorCodeOutput=on  ModelName=ROPOD_4Wheel_kinb_cntr  BlockId=ParamGet_ROPOD_4Wheel_kinb_cntr_1102
      settings: SourceProductName=Robotics System Toolbox  SourceProductBaseCode=RO
  Get Parameter5 : robotlib/Get Parameter  SourceLibraryInfo=This block requires Robotics System Toolbox  ParameterSource=Specify your own  ParameterName=/base_kin_model/xpos_SW2  ParameterType=double  ParameterMaxArrayLength=16  ParameterInitialValue=ropod_kinmodel_param.C_SW(3)  SampleTime=Tsp  ShowErrorCodeOutput=on  ModelName=ROPOD_4Wheel_kinb_cntr  BlockId=ParamGet_ROPOD_4Wheel_kinb_cntr_1103
      settings: SourceProductName=Robotics System Toolbox  SourceProductBaseCode=RO
  Get Parameter6 : robotlib/Get Parameter  SourceLibraryInfo=This block requires Robotics System Toolbox  ParameterSource=Specify your own  ParameterName=/base_kin_model/ypos_SW2  ParameterType=double  ParameterMaxArrayLength=16  ParameterInitialValue=ropod_kinmodel_param.C_SW(4)  SampleTime=Tsp  ShowErrorCodeOutput=on  ModelName=ROPOD_4Wheel_kinb_cntr  BlockId=ParamGet_ROPOD_4Wheel_kinb_cntr_1104
      settings: SourceProductName=Robotics System Toolbox  SourceProductBaseCode=RO
  Get Parameter7 : robotlib/Get Parameter  SourceLibraryInfo=This block requires Robotics System Toolbox  ParameterSource=Specify your own  ParameterName=/base_kin_model/xpos_SW3  ParameterType=double  ParameterMaxArrayLength=16  ParameterInitialValue=ropod_kinmodel_param.C_SW(5)  SampleTime=Tsp  ShowErrorCodeOutput=on  ModelName=ROPOD_4Wheel_kinb_cntr  BlockId=ParamGet_ROPOD_4Wheel_kinb_cntr_1110
      settings: SourceProductName=Robotics System Toolbox  SourceProductBaseCode=RO
  Get Parameter8 : robotlib/Get Parameter  SourceLibraryInfo=This block requires Robotics System Toolbox  ParameterSource=Specify your own  ParameterName=/base_kin_model/ypos_SW3  ParameterType=double  ParameterMaxArrayLength=16  ParameterInitialValue=ropod_kinmodel_param.C_SW(6)  SampleTime=Tsp  ShowErrorCodeOutput=on  ModelName=ROPOD_4Wheel_kinb_cntr  BlockId=ParamGet_ROPOD_4Wheel_kinb_cntr_1111
      settings: SourceProductName=Robotics System Toolbox  SourceProductBaseCode=RO
  Get Parameter9 : robotlib/Get Parameter  SourceLibraryInfo=This block requires Robotics System Toolbox  ParameterSource=Specify your own  ParameterName=/base_kin_model/xpos_SW4  ParameterType=double  ParameterMaxArrayLength=16  ParameterInitialValue=ropod_kinmodel_param.C_SW(7)  SampleTime=Tsp  ShowErrorCodeOutput=on  ModelName=ROPOD_4Wheel_kinb_cntr  BlockId=ParamGet_ROPOD_4Wheel_kinb_cntr_1112
      settings: SourceProductName=Robotics System Toolbox  SourceProductBaseCode=RO
  Mux : Mux  Inputs=18
  Terminator{,1..17} (18 alike) : Terminator
  ropod_kin_param : Outport
  wires:
  Mux/1 -> ropod_kin_param/1
  Get Parameter/2 -> Terminator/1
  Get Parameter13/1 -> Mux/4
  Get Parameter15/2 -> Terminator15/1
  Get Parameter14/2 -> Terminator14/1
  Get Parameter16/1 -> Mux/7
  Get Parameter15/1 -> Mux/6
  Get Parameter11/1 -> Mux/2
  Get Parameter11/2 -> Terminator11/1
  Get Parameter16/2 -> Terminator16/1
  Get Parameter12/2 -> Terminator12/1
  Get Parameter12/1 -> Mux/3
  Get Parameter/1 -> Mux/1
  Get Parameter17/2 -> Terminator17/1
  Get Parameter13/2 -> Terminator13/1
  Get Parameter17/1 -> Mux/8
  Get Parameter14/1 -> Mux/5
  Get Parameter2/2 -> Terminator2/1
  Get Parameter2/1 -> Mux/10
  Get Parameter1/1 -> Mux/9
  Get Parameter1/2 -> Terminator1/1
  Get Parameter6/2 -> Terminator6/1
  Get Parameter6/1 -> Mux/14
  Get Parameter3/1 -> Mux/11
  Get Parameter5/2 -> Terminator5/1
  Get Parameter5/1 -> Mux/13
  Get Parameter4/1 -> Mux/12
  Get Parameter3/2 -> Terminator3/1
  Get Parameter4/2 -> Terminator4/1
  Get Parameter10/1 -> Mux/18
  Get Parameter10/2 -> Terminator10/1
  Get Parameter8/2 -> Terminator8/1
  Get Parameter7/2 -> Terminator7/1
  Get Parameter9/2 -> Terminator9/1
  Get Parameter7/1 -> Mux/15
  Get Parameter8/1 -> Mux/16
  Get Parameter9/1 -> Mux/17

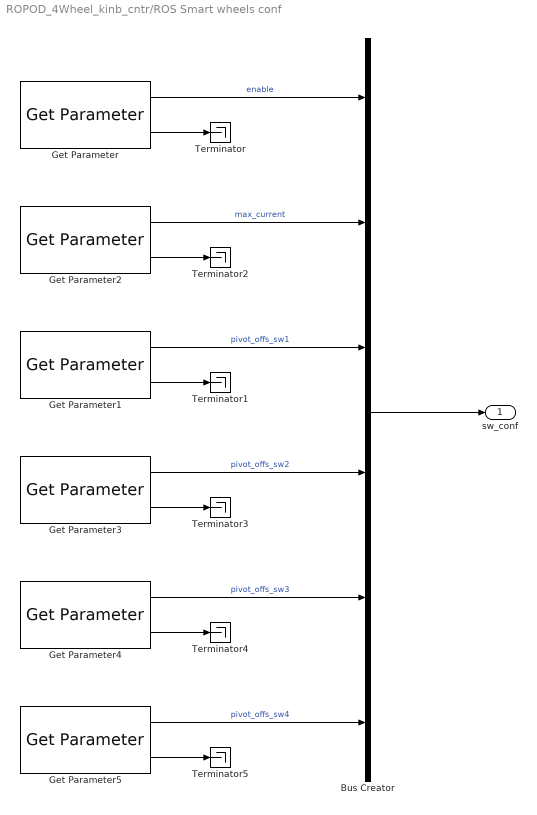
== system ROPOD_4Wheel_kinb_cntr/ROS Smart wheels conf ==
  Bus Creator : BusCreator  Inputs=6
  Get Parameter : robotlib/Get Parameter  SourceLibraryInfo=This block requires Robotics System Toolbox  ParameterSource=Specify your own  ParameterName=/smart_wheels/enable  ParameterType=double  ParameterMaxArrayLength=16  ParameterInitialValue=sw_ini_enable  SampleTime=Tsp  ShowErrorCodeOutput=on  ModelName=ROPOD_4Wheel_kinb_cntr  BlockId=ParamGet_ROPOD_4Wheel_kinb_cntr_542
      settings: SourceProductName=Robotics System Toolbox  SourceProductBaseCode=RO
  Get Parameter1 : robotlib/Get Parameter  SourceLibraryInfo=This block requires Robotics System Toolbox  ParameterSource=Specify your own  ParameterName=/smart_wheels/pivot_offs_sw1  ParameterType=double  ParameterMaxArrayLength=16  ParameterInitialValue=pivot_offs_sws(1)  SampleTime=Tsp  ShowErrorCodeOutput=on  ModelName=ROPOD_4Wheel_kinb_cntr  BlockId=ParamGet_ROPOD_4Wheel_kinb_cntr_1130
      settings: SourceProductName=Robotics System Toolbox  SourceProductBaseCode=RO
  Get Parameter2 : robotlib/Get Parameter  SourceLibraryInfo=This block requires Robotics System Toolbox  ParameterSource=Specify your own  ParameterName=/smart_wheels/max_current  ParameterType=double  ParameterMaxArrayLength=16  ParameterInitialValue=max_sw_current  SampleTime=Tsp  ShowErrorCodeOutput=on  ModelName=ROPOD_4Wheel_kinb_cntr  BlockId=ParamGet_ROPOD_4Wheel_kinb_cntr_544
      settings: SourceProductName=Robotics System Toolbox  SourceProductBaseCode=RO
  Get Parameter3 : robotlib/Get Parameter  SourceLibraryInfo=This block requires Robotics System Toolbox  ParameterSource=Specify your own  ParameterName=/smart_wheels/pivot_offs_sw2  ParameterType=double  ParameterMaxArrayLength=16  ParameterInitialValue=pivot_offs_sws(2)  SampleTime=Tsp  ShowErrorCodeOutput=on  ModelName=ROPOD_4Wheel_kinb_cntr  BlockId=ParamGet_ROPOD_4Wheel_kinb_cntr_1132
      settings: SourceProductName=Robotics System Toolbox  SourceProductBaseCode=RO
  Get Parameter4 : robotlib/Get Parameter  SourceLibraryInfo=This block requires Robotics System Toolbox  ParameterSource=Specify your own  ParameterName=/smart_wheels/pivot_offs_sw3  ParameterType=double  ParameterMaxArrayLength=16  ParameterInitialValue=pivot_offs_sws(3)  SampleTime=Tsp  ShowErrorCodeOutput=on  ModelName=ROPOD_4Wheel_kinb_cntr  BlockId=ParamGet_ROPOD_4Wheel_kinb_cntr_1134
      settings: SourceProductName=Robotics System Toolbox  SourceProductBaseCode=RO
  Get Parameter5 : robotlib/Get Parameter  SourceLibraryInfo=This block requires Robotics System Toolbox  ParameterSource=Specify your own  ParameterName=/smart_wheels/pivot_offs_sw4  ParameterType=double  ParameterMaxArrayLength=16  ParameterInitialValue=pivot_offs_sws(4)  SampleTime=Tsp  ShowErrorCodeOutput=on  ModelName=ROPOD_4Wheel_kinb_cntr  BlockId=ParamGet_ROPOD_4Wheel_kinb_cntr_1136
      settings: SourceProductName=Robotics System Toolbox  SourceProductBaseCode=RO
  Terminator{,1..5} (6 alike) : Terminator
  sw_conf : Outport
  wires:
  Get Parameter/2 -> Terminator/1
  Get Parameter/1 -> Bus Creator/1  "enable"
  Bus Creator/1 -> sw_conf/1
  Get Parameter2/2 -> Terminator2/1
  Get Parameter2/1 -> Bus Creator/2  "max_current"
  Get Parameter1/1 -> Bus Creator/3  "pivot_offs_sw1"
  Get Parameter1/2 -> Terminator1/1
  Get Parameter3/2 -> Terminator3/1
  Get Parameter3/1 -> Bus Creator/4  "pivot_offs_sw2"
  Get Parameter4/2 -> Terminator4/1
  Get Parameter4/1 -> Bus Creator/5  "pivot_offs_sw3"
  Get Parameter5/2 -> Terminator5/1
  Get Parameter5/1 -> Bus Creator/6  "pivot_offs_sw4"

== system ROPOD_4Wheel_kinb_cntr/ROS Smart wheels conf1 ==
  Bus Creator : BusCreator  Inputs=2
  enable : Constant
  max_current : Constant  Value=max_sw_current
  sw_conf : Outport
  wires:
  enable/1 -> Bus Creator/1  "enable"
  Bus Creator/1 -> sw_conf/1
  max_current/1 -> Bus Creator/2  "max_current"

== system ROPOD_4Wheel_kinb_cntr/ROS base conf ==
  Bus Creator : BusCreator  Inputs=4
  Get Parameter : robotlib/Get Parameter  SourceLibraryInfo=This block requires Robotics System Toolbox  ParameterSource=Specify your own  ParameterName=/base_conf/max_acc_xy  ParameterType=double  ParameterMaxArrayLength=16  ParameterInitialValue=max_ropod_acc_xy  SampleTime=Tsp  ShowErrorCodeOutput=on  ModelName=ROPOD_4Wheel_kinb_cntr  BlockId=ParamGet_ROPOD_4Wheel_kinb_cntr_551
      settings: SourceProductName=Robotics System Toolbox  SourceProductBaseCode=RO
  Get Parameter1 : robotlib/Get Parameter  SourceLibraryInfo=This block requires Robotics System Toolbox  ParameterSource=Specify your own  ParameterName=/base_conf/max_vel_xy  ParameterType=double  ParameterMaxArrayLength=16  ParameterInitialValue=max_ropod_vel_xy  SampleTime=Tsp  ShowErrorCodeOutput=on  ModelName=ROPOD_4Wheel_kinb_cntr  BlockId=ParamGet_ROPOD_4Wheel_kinb_cntr_552
      settings: SourceProductName=Robotics System Toolbox  SourceProductBaseCode=RO
  Get Parameter2 : robotlib/Get Parameter  SourceLibraryInfo=This block requires Robotics System Toolbox  ParameterSource=Specify your own  ParameterName=/base_conf/max_acc_theta  ParameterType=double  ParameterMaxArrayLength=16  ParameterInitialValue=max_ropod_acc_theta  SampleTime=Tsp  ShowErrorCodeOutput=on  ModelName=ROPOD_4Wheel_kinb_cntr  BlockId=ParamGet_ROPOD_4Wheel_kinb_cntr_664
      settings: SourceProductName=Robotics System Toolbox  SourceProductBaseCode=RO
  Get Parameter3 : robotlib/Get Parameter  SourceLibraryInfo=This block requires Robotics System Toolbox  ParameterSource=Specify your own  ParameterName=/base_conf/max_vel_theta  ParameterType=double  ParameterMaxArrayLength=16  ParameterInitialValue=max_ropod_vel_theta  SampleTime=Tsp  ShowErrorCodeOutput=on  ModelName=ROPOD_4Wheel_kinb_cntr  BlockId=ParamGet_ROPOD_4Wheel_kinb_cntr_665
      settings: SourceProductName=Robotics System Toolbox  SourceProductBaseCode=RO
  Terminator{,1..3} (4 alike) : Terminator
  base_conf : Outport
  wires:
  Get Parameter/2 -> Terminator/1
  Get Parameter1/2 -> Terminator1/1
  Get Parameter/1 -> Bus Creator/2  "max_acc_xy"
  Get Parameter1/1 -> Bus Creator/1  "max_vel_xy"
  Bus Creator/1 -> base_conf/1
  Get Parameter2/2 -> Terminator2/1
  Get Parameter2/1 -> Bus Creator/4  "max_acc_theta"
  Get Parameter3/1 -> Bus Creator/3  "max_vel_theta"
  Get Parameter3/2 -> Terminator3/1

== system ROPOD_4Wheel_kinb_cntr/ROS base conf1 ==
  Bus Creator : BusCreator  Inputs=4
  Constant1 : Constant  Value=max_ropod_vel_xy
  Constant2 : Constant  Value=max_ropod_acc_xy
  Constant3 : Constant  Value=max_ropod_vel_theta
  Constant4 : Constant  Value=max_ropod_acc_theta
  base_conf : Outport
  wires:
  Constant4/1 -> Bus Creator/4  "max_acc_theta"
  Constant1/1 -> Bus Creator/1  "max_vel_xy"
  Constant3/1 -> Bus Creator/3  "max_vel_theta"
  Bus Creator/1 -> base_conf/1
  Constant2/1 -> Bus Creator/2  "max_acc_xy"

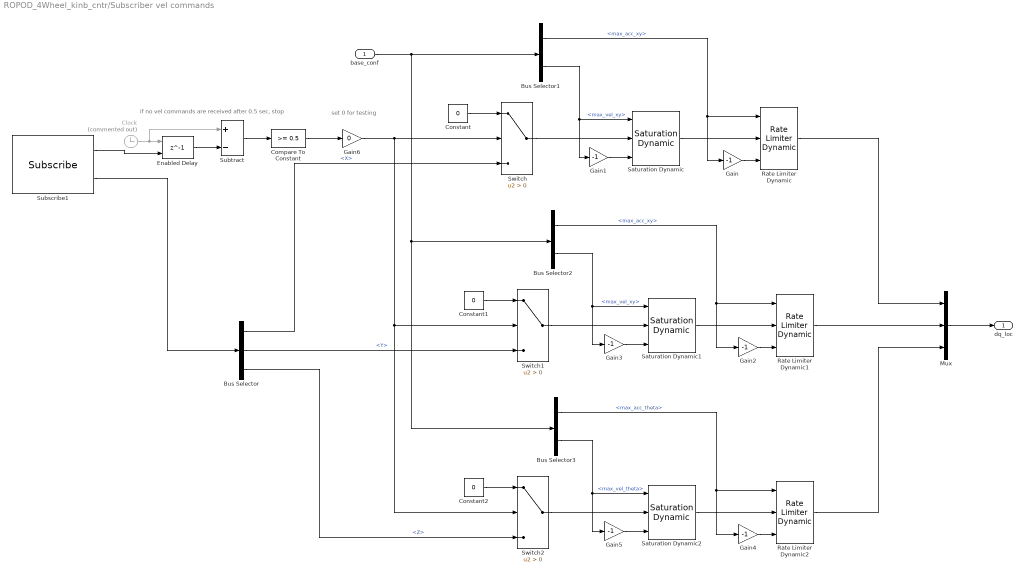
== system ROPOD_4Wheel_kinb_cntr/Subscriber vel commands ==
  note: set 0 for testing
  note: if no vel commands are received after 0.5 sec, stop
  base_conf : Inport
  Bus Selector : BusSelector  OutputSignals=Linear.X,Linear.Y,Angular.Z
  Bus Selector1 : BusSelector  OutputSignals=max_acc_xy,max_vel_xy
  Bus Selector2 : BusSelector  OutputSignals=max_acc_xy,max_vel_xy
  Bus Selector3 : BusSelector  OutputSignals=max_acc_theta,max_vel_theta
  Clock : Clock  Commented=on
  Compare To Constant : simulink/Logic and Bit Operations/Compare To Constant  relop=>=  const=0.5  OutDataTypeStr=boolean
  Constant : Constant  Value=0
  Constant1 : Constant  Value=0
  Constant2 : Constant  Value=0
  Enabled Delay : Delay  DelayLength=1  ShowEnablePort=on
      settings: InputPortMap=u0,e6
  Gain{,1..5} (6 alike) : Gain  Gain=-1
  Gain6 : Gain  Gain=0
  Mux : Mux  Inputs=3
  Rate Limiter Dynamic : simulink/Discontinuities/Rate Limiter Dynamic
      settings: SourceProductName=Simulink
  Rate Limiter Dynamic1 : simulink/Discontinuities/Rate Limiter Dynamic
      settings: SourceProductName=Simulink
  Rate Limiter Dynamic2 : simulink/Discontinuities/Rate Limiter Dynamic
      settings: SourceProductName=Simulink
  Saturation Dynamic : simulink/Discontinuities/Saturation Dynamic  OutMin=[]  OutMax=[]  OutDataTypeStr=Inherit: Same as second input  OutDataType=fixdt(1, 16)  OutScaling=2^-10  DoSatur=off
  Saturation Dynamic1 : simulink/Discontinuities/Saturation Dynamic  OutMin=[]  OutMax=[]  OutDataTypeStr=Inherit: Same as second input  OutDataType=fixdt(1, 16)  OutScaling=2^-10  DoSatur=off
  Saturation Dynamic2 : simulink/Discontinuities/Saturation Dynamic  OutMin=[]  OutMax=[]  OutDataTypeStr=Inherit: Same as second input  OutDataType=fixdt(1, 16)  OutScaling=2^-10  DoSatur=off
  Subscribe1 : robotlib/Subscribe  SourceLibraryInfo=This block requires Robotics System Toolbox  topicSource=Specify your own  topic=/pico/cmd_vel  messageType=geometry_msgs/Twist  sampleTime=Ts_rost  messageQueueLength=5
      settings: SourceProductBaseCode=RO
  Subtract : Sum  Inputs=+-
  Switch : Switch  Criteria=u2 > Threshold
  Switch1 : Switch  Criteria=u2 > Threshold
  Switch2 : Switch  Criteria=u2 > Threshold
  dq_loc : Outport
  wires:
  Bus Selector/1 -> Switch/3  "<X>"
  Subscribe1/2 -> Bus Selector/1
  Subscribe1/1 -> Enabled Delay/2
  Clock/1 -> Subtract/1, Enabled Delay/1
  Enabled Delay/1 -> Subtract/2
  Subtract/1 -> Compare To Constant/1
  Constant/1 -> Switch/1
  Gain/1 -> Rate Limiter Dynamic/3
  Switch/1 -> Saturation Dynamic/2
  Gain1/1 -> Saturation Dynamic/3
  Saturation Dynamic/1 -> Rate Limiter Dynamic/2
  Switch1/1 -> Saturation Dynamic1/2
  Gain3/1 -> Saturation Dynamic1/3
  Constant1/1 -> Switch1/1
  Bus Selector/2 -> Switch1/3  "<Y>"
  Gain2/1 -> Rate Limiter Dynamic1/3
  Saturation Dynamic1/1 -> Rate Limiter Dynamic1/2
  Bus Selector2/1 -> Rate Limiter Dynamic1/1, Gain2/1  "<max_acc_xy>"
  Bus Selector2/2 -> Saturation Dynamic1/1, Gain3/1  "<max_vel_xy>"
  Bus Selector3/1 -> Rate Limiter Dynamic2/1, Gain4/1  "<max_acc_theta>"
  Saturation Dynamic2/1 -> Rate Limiter Dynamic2/2
  base_conf/1 -> Bus Selector3/1, Bus Selector2/1, Bus Selector1/1
  Switch2/1 -> Saturation Dynamic2/2
  Constant2/1 -> Switch2/1
  Bus Selector/3 -> Switch2/3  "<Z>"
  Gain5/1 -> Saturation Dynamic2/3
  Gain4/1 -> Rate Limiter Dynamic2/3
  Compare To Constant/1 -> Gain6/1
  Bus Selector3/2 -> Saturation Dynamic2/1, Gain5/1  "<max_vel_theta>"
  Mux/1 -> dq_loc/1
  Rate Limiter Dynamic/1 -> Mux/1
  Rate Limiter Dynamic1/1 -> Mux/2
  Rate Limiter Dynamic2/1 -> Mux/3
  Bus Selector1/2 -> Saturation Dynamic/1, Gain1/1  "<max_vel_xy>"
  Bus Selector1/1 -> Rate Limiter Dynamic/1, Gain/1  "<max_acc_xy>"
  Gain6/1 -> Switch2/2, Switch1/2, Switch/2
